simulink model "Real_three_Medusa_CPF_Event_Communication_For_Test"  (Simulink 8.7)
settings: Solver=ode45  StartTime=0.0  StopTime=400  FixedStep=Ts  RelTol=1e-3
values from neighbouring files (symbols this model uses):
  L = 50    [initialization_3vehicles.m]
  m1 = 0    [initialization_3vehicles.m]
  m2 = 0    [initialization_3vehicles.m]
  m3 = 0    [initialization_3vehicles.m]
  R = 12    [initialization_3vehicles.m]
  Ts = 0.01    [initialization_3vehicles.m]
libraries: Mylibrary x6
settings Model: Creator=hung  LastModifiedBy=hung
settings DebuggingCC: SolverPrmCheckMsg=warning  StateNameClashWarn=warning

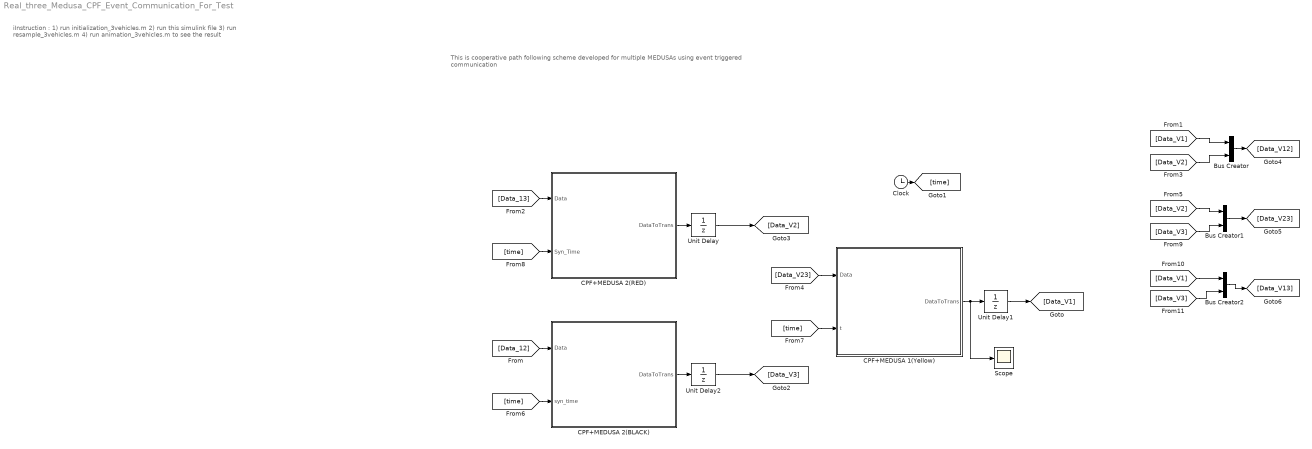
== system Real_three_Medusa_CPF_Event_Communication_For_Test ==
  note: iInstruction :
      |
      | 1) run initialization_3vehicles.m
      | 2) run this simulink file
      | 3) run resample_3vehicles.m
      | 4) run animation_3vehicles.m
      | to see the result
  note: This is cooperative path following scheme developed for multiple MEDUSAs using event triggered communication
  Bus Creator : BusCreator  Inputs=2
  Bus Creator1 : BusCreator  Inputs=2
  Bus Creator2 : BusCreator  Inputs=2
  CPF+MEDUSA 1(Yellow) : Subsystem  Priority=2  TreatAsAtomicUnit=on  mask{Vehicle_Index=1}
      mask Display: image('MEDUSA_YELLOW.png');
  CPF+MEDUSA 2(BLACK) : Subsystem  Priority=2  TreatAsAtomicUnit=on  mask{Vehicle_Index=3}
      mask Display: image('MEDUSA_BLACK.png');
  CPF+MEDUSA 2(RED) : Subsystem  Priority=2  TreatAsAtomicUnit=on  mask{Vehicle_Index=2}
      mask Display: image('MEDUSA_RED.png');
  Clock : Clock
  Scope : Scope
  Unit Delay : UnitDelay  SampleTime=Ts
  Unit Delay1 : UnitDelay  SampleTime=Ts
  Unit Delay2 : UnitDelay  SampleTime=Ts
  wires:
  Clock/1 -> [time]
  CPF+MEDUSA 1(Yellow)/1(DataToTrans) -> Scope/1, Unit Delay1/1
  [Data_12] -> CPF+MEDUSA 2(BLACK)/1(Data)
  CPF+MEDUSA 2(BLACK)/1(DataToTrans) -> Unit Delay2/1
  CPF+MEDUSA 2(RED)/1(DataToTrans) -> Unit Delay/1
  [Data_13] -> CPF+MEDUSA 2(RED)/1(Data)
  [Data_V23] -> CPF+MEDUSA 1(Yellow)/1(Data)
  [time] -> CPF+MEDUSA 2(BLACK)/2(syn_time)
  [time] -> CPF+MEDUSA 1(Yellow)/2(t)
  [time] -> CPF+MEDUSA 2(RED)/2(Syn_Time)
  Unit Delay/1 -> [Data_V2]
  Unit Delay1/1 -> [Data_V1]
  Unit Delay2/1 -> [Data_V3]
  Bus Creator/1 -> [Data_V12]
  [Data_V2] -> Bus Creator/2
  [Data_V1] -> Bus Creator/1
  Bus Creator1/1 -> [Data_V23]
  [Data_V2] -> Bus Creator1/1
  [Data_V3] -> Bus Creator1/2
  Bus Creator2/1 -> [Data_V13]
  [Data_V1] -> Bus Creator2/1
  [Data_V3] -> Bus Creator2/2

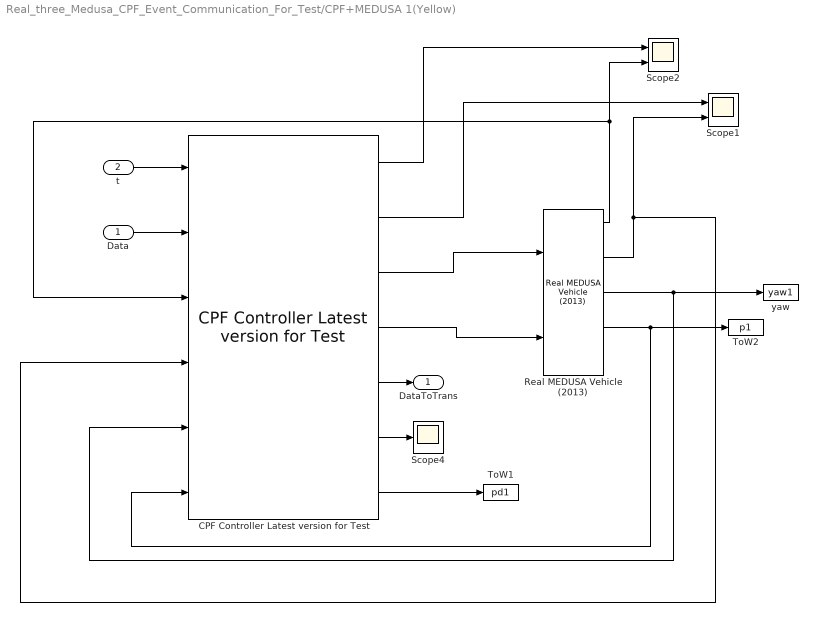
== system Real_three_Medusa_CPF_Event_Communication_For_Test/CPF+MEDUSA 1(Yellow) ==
  Data : Inport
  t : Inport  Port=2
  " Real MEDUSA Vehicle (2013)" : Mylibrary/ Real MEDUSA Vehicle (2013)  x0=x10  y0=y10  yaw0=yaw10  u0=0  v0=0  r0=0  dist_u=0  dist_v=0  dist_r=0  Vcx=Vcx  Vcy=Vcy
  CPF Controller Latest version for Test : Mylibrary/CPF Controller Latest version for Test  vp=vp  L=L  m=m1  d=d1  R=R  tau_bar=tau_bar  Mode=Mode  T_Trigger=T_Trigger  Parameter9=epsilon  V_Id=3
  Scope1 : Scope  NumInputPorts=2
  Scope2 : Scope  NumInputPorts=2
  Scope4 : Scope
  ToW1 : ToWorkspace  VariableName=pd1  SampleTime=Ts
  ToW2 : ToWorkspace  VariableName=p1  SampleTime=Ts
  yaw : ToWorkspace  VariableName=yaw1  SampleTime=Ts
  DataToTrans : Outport
  wires:
  " Real MEDUSA Vehicle (2013)"/3 -> CPF Controller Latest version for Test/5, yaw/1
  " Real MEDUSA Vehicle (2013)"/4 -> CPF Controller Latest version for Test/6, ToW2/1
  t/1 -> CPF Controller Latest version for Test/1
  Data/1 -> CPF Controller Latest version for Test/2
  CPF Controller Latest version for Test/5 -> DataToTrans/1
  CPF Controller Latest version for Test/6 -> Scope4/1
  CPF Controller Latest version for Test/7 -> ToW1/1
  CPF Controller Latest version for Test/3 -> " Real MEDUSA Vehicle (2013)"/1
  CPF Controller Latest version for Test/4 -> " Real MEDUSA Vehicle (2013)"/2
  " Real MEDUSA Vehicle (2013)"/2 -> Scope1/2, CPF Controller Latest version for Test/4
  " Real MEDUSA Vehicle (2013)"/1 -> CPF Controller Latest version for Test/3, Scope2/2
  CPF Controller Latest version for Test/2 -> Scope1/1
  CPF Controller Latest version for Test/1 -> Scope2/1

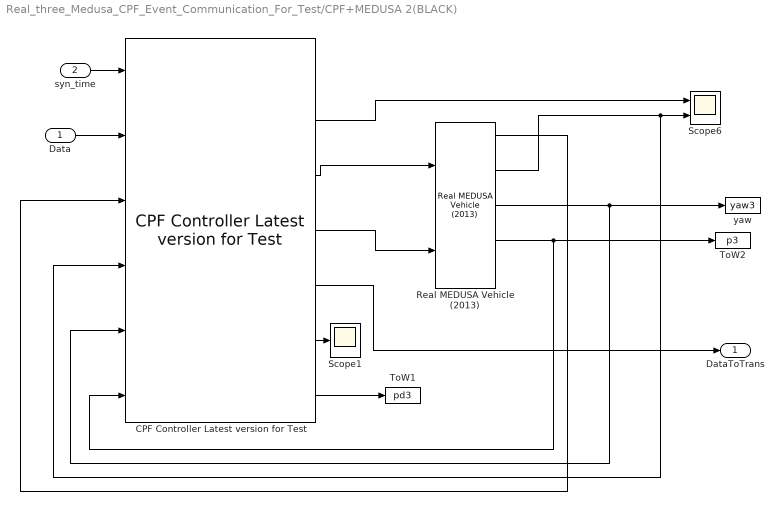
== system Real_three_Medusa_CPF_Event_Communication_For_Test/CPF+MEDUSA 2(BLACK) ==
  Data : Inport
  syn_time : Inport  Port=2
  " Real MEDUSA Vehicle (2013)" : Mylibrary/ Real MEDUSA Vehicle (2013)  x0=x20  y0=y20  yaw0=yaw20  u0=0  v0=0  r0=0  dist_u=0  dist_v=0  dist_r=0  Vcx=Vcx  Vcy=Vcy
  CPF Controller Latest version for Test : Mylibrary/CPF Controller Latest version for Test  vp=vp  L=L  m=m3  d=d3  R=R  tau_bar=tau_bar  Mode=Mode  T_Trigger=T_Trigger  Parameter9=epsilon  V_Id=3
  Scope1 : Scope
  Scope6 : Scope  NumInputPorts=2
  ToW1 : ToWorkspace  VariableName=pd3  SampleTime=Ts
  ToW2 : ToWorkspace  VariableName=p3  SampleTime=Ts
  yaw : ToWorkspace  VariableName=yaw3  SampleTime=Ts
  DataToTrans : Outport
  wires:
  " Real MEDUSA Vehicle (2013)"/3 -> CPF Controller Latest version for Test/5, yaw/1
  " Real MEDUSA Vehicle (2013)"/4 -> CPF Controller Latest version for Test/6, ToW2/1
  syn_time/1 -> CPF Controller Latest version for Test/1
  CPF Controller Latest version for Test/5 -> DataToTrans/1
  CPF Controller Latest version for Test/3 -> " Real MEDUSA Vehicle (2013)"/1
  Data/1 -> CPF Controller Latest version for Test/2
  CPF Controller Latest version for Test/7 -> ToW1/1
  CPF Controller Latest version for Test/4 -> " Real MEDUSA Vehicle (2013)"/2
  CPF Controller Latest version for Test/6 -> Scope1/1
  CPF Controller Latest version for Test/2 -> Scope6/1
  " Real MEDUSA Vehicle (2013)"/2 -> CPF Controller Latest version for Test/4, Scope6/2
  " Real MEDUSA Vehicle (2013)"/1 -> CPF Controller Latest version for Test/3

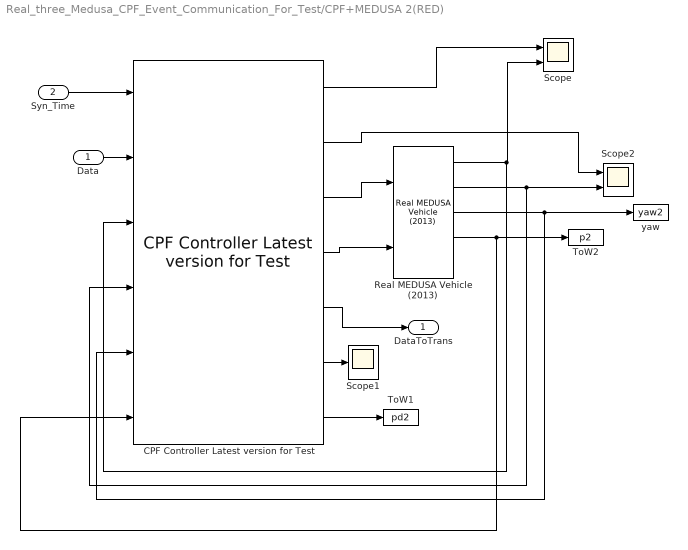
== system Real_three_Medusa_CPF_Event_Communication_For_Test/CPF+MEDUSA 2(RED) ==
  Data : Inport
  Syn_Time : Inport  Port=2
  " Real MEDUSA Vehicle (2013)" : Mylibrary/ Real MEDUSA Vehicle (2013)  x0=x30  y0=y30  yaw0=yaw30  u0=0  v0=0  r0=0  dist_u=0  dist_v=0  dist_r=0  Vcx=Vcx  Vcy=Vcy
  CPF Controller Latest version for Test : Mylibrary/CPF Controller Latest version for Test  vp=vp  L=L  m=m2  d=d2  R=R  tau_bar=tau_bar  Mode=Mode  T_Trigger=T_Trigger  Parameter9=epsilon  V_Id=1
  Scope : Scope  NumInputPorts=2
  Scope1 : Scope
  Scope2 : Scope  NumInputPorts=2
  ToW1 : ToWorkspace  VariableName=pd2  SampleTime=Ts
  ToW2 : ToWorkspace  VariableName=p2  SampleTime=Ts
  yaw : ToWorkspace  VariableName=yaw2  SampleTime=Ts
  DataToTrans : Outport
  wires:
  " Real MEDUSA Vehicle (2013)"/1 -> CPF Controller Latest version for Test/3, Scope/2
  " Real MEDUSA Vehicle (2013)"/4 -> CPF Controller Latest version for Test/6, ToW2/1
  " Real MEDUSA Vehicle (2013)"/3 -> CPF Controller Latest version for Test/5, yaw/1
  " Real MEDUSA Vehicle (2013)"/2 -> CPF Controller Latest version for Test/4, Scope2/2
  CPF Controller Latest version for Test/3 -> " Real MEDUSA Vehicle (2013)"/1
  CPF Controller Latest version for Test/5 -> DataToTrans/1
  Data/1 -> CPF Controller Latest version for Test/2
  Syn_Time/1 -> CPF Controller Latest version for Test/1
  CPF Controller Latest version for Test/7 -> ToW1/1
  CPF Controller Latest version for Test/4 -> " Real MEDUSA Vehicle (2013)"/2
  CPF Controller Latest version for Test/1 -> Scope/1
  CPF Controller Latest version for Test/6 -> Scope1/1
  CPF Controller Latest version for Test/2 -> Scope2/1
